simulink model "interpolation_nD_TestGen19"  (R2017b)
settings: Solver=FixedStepDiscrete  StartTime=0.0  StopTime=10.0  RelTol=1e-3
settings Model: Creator=ktrinh  LastModifiedBy=ktrinh
settings DebuggingCC: ParameterOverflowMsg=none

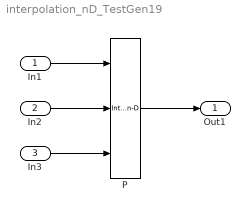
== system interpolation_nD_TestGen19 ==
  In1 : Inport  OutMin=0  OutMax=2  PortDimensions=3
  In2 : Inport  Port=2  OutMin=-0.5  OutMax=1.5
  In3 : Inport  Port=3  OutMin=0  OutMax=5
  P : Interpolation_n-D  Table=[12.7730979567253 27.4147441452008 44.727386075552 13.7905308176609 26.1531162250115;32.6405642155552 41.4259885127561 107.303073329967 17.675701262502 5.83955255452587]  InterpMethod=Flat  ExtrapMethod=Clip  ValidIndexMayReachLast=on  NumSelectionDims=1  OutDataTypeStr=uint32  InternalRulePriority=Speed  RndMeth=Simplest  SaturateOnIntegerOverflow=on
      settings: InputPortMap=u0,u1,u2
  Out1 : Outport
  wires:
  In1/1 -> P/1
  In2/1 -> P/2
  In3/1 -> P/3
  P/1 -> Out1/1
